simulink model "logistic"  (R2024b)
settings: Solver=VariableStepAuto  StartTime=0.0  StopTime=10.0  RelTol=1e-3
settings Model: Creator=Botló  LastModifiedBy=Botló

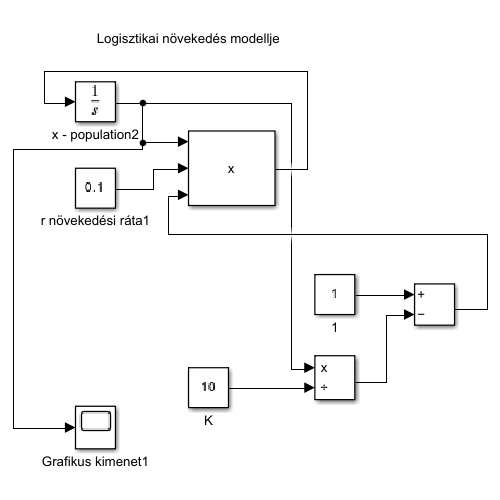
[thumbnail: Simulink's stored preview of the top-level diagram]
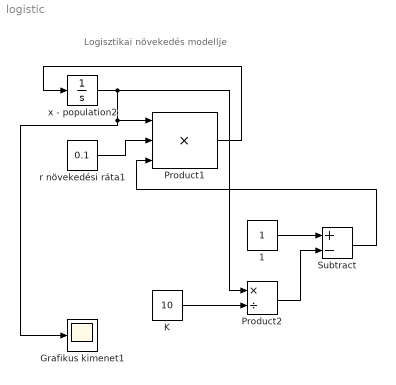
== system logistic ==
  note: Logisztikai növekedés modellje
  1 : Constant
  Grafikus kimenet1 : Scope
  K : Constant  Value=10
  Product1 : Product  Inputs=3
  Product2 : Product  Inputs=*/
  Subtract : Sum  Inputs=+-
  r növekedési ráta1 : Constant  Value=0.1
  x - population2 : Integrator  InitialCondition=1
  wires:
  Product2/1 -> Subtract/2
  1/1 -> Subtract/1
  Subtract/1 -> Product1/3
  r növekedési ráta1/1 -> Product1/2
  x - population2/1 -> Product2/1, Grafikus kimenet1/1, Product1/1
  Product1/1 -> x - population2/1
  K/1 -> Product2/2
